simulink subsystem "pitchYawInnerLoop"  (R2026a)
settings: Solver=VariableStepAuto
values from neighbouring files (symbols this model uses):
  innerLoopParams = 180.0    [controllerParams.sldd]
libraries: slctrl_autotuning x1
settings Model: DataDictionary=controllerParams.sldd  EnableAccessToBaseWorkspace=off  Creator=maxhu  LastModifiedBy=maxhu

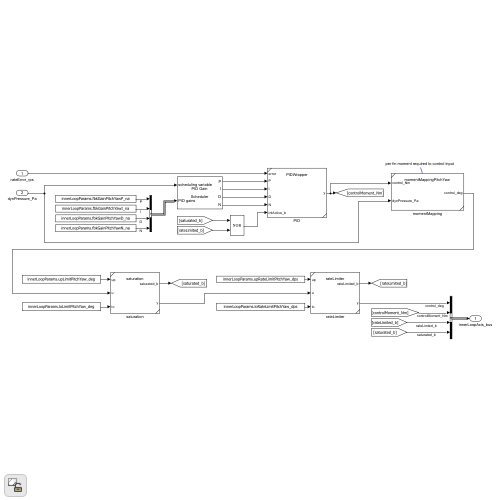
[thumbnail: Simulink's stored preview of the top-level diagram]
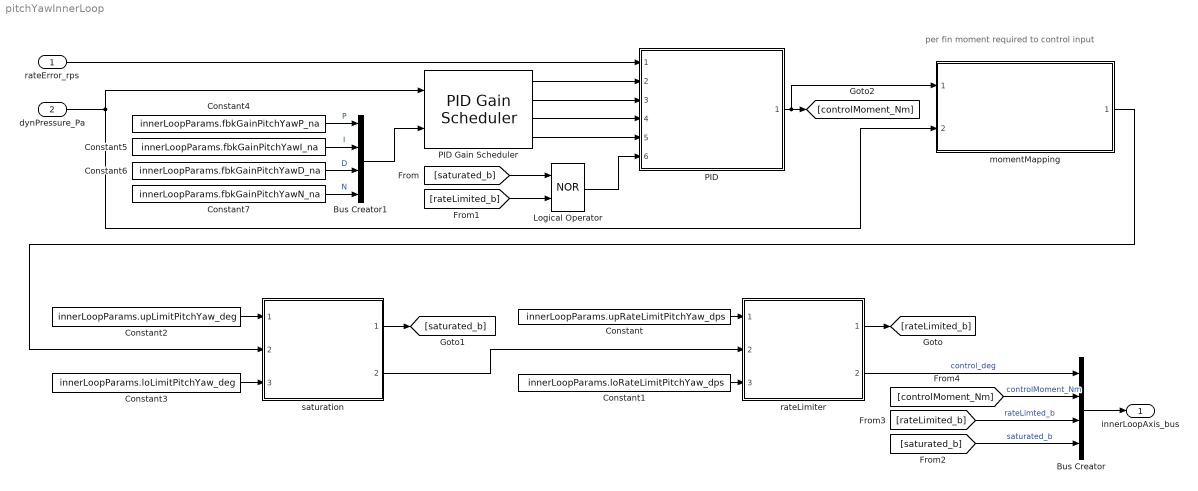
== system pitchYawInnerLoop ==
  note: per fin moment required to control input
  rateError_rps : Inport
  dynPressure_Pa : Inport  Port=2
  Bus Creator : BusCreator  Inputs=4
  Bus Creator1 : BusCreator  Inputs=4
  Constant : Constant  Value=innerLoopParams.upRateLimitPitchYaw_dps
  Constant1 : Constant  Value=innerLoopParams.loRateLimitPitchYaw_dps
  Constant2 : Constant  Value=innerLoopParams.upLimitPitchYaw_deg
  Constant3 : Constant  Value=innerLoopParams.loLimitPitchYaw_deg
  Constant4 : Constant  Value=innerLoopParams.fbkGainPitchYawP_na
  Constant5 : Constant  Value=innerLoopParams.fbkGainPitchYawI_na
  Constant6 : Constant  Value=innerLoopParams.fbkGainPitchYawD_na
  Constant7 : Constant  Value=innerLoopParams.fbkGainPitchYawN_na
  Logical Operator : Logic  Operator=NOR  AllPortsSameDT=off  OutDataTypeStr=boolean
  PID : Subsystem  ReferencedSubsystem=PIDWrapper
  PID Gain Scheduler : slctrl_autotuning/PID Gain Scheduler  InstantiateOnLoad=on  ControllerType=PIDN  BPsInGainArray=off  UseTwoSchedulingVariables=off  GainArrayBreakpoints=innerLoopParams.fbkGainBreakpoints_Pa  GainArrayBreakpoints2=[1 2 3 4]  NumBreakpoints=3  NumBreakpoints2=4  UseExternalBreakpoints=off  GainSourceMethod=Input to block  StoreGainsPParamName=PGain  StoreGainsIParamName=IGain  StoreGainsDParamName=DGain  StoreGainsNParamName=NGain  BlockDataType=Double  PGainLookUpMeth=Interpolation-Use End Values  IGainLookUpMeth=Interpolation-Use End Values  DGainLookUpMeth=Interpolation-Use End Values  NGainLookUpMeth=Interpolation-Use End Values  DoSatur=off  BreakpointSourceLookupVariant=InternalBPs  GainSourceVariant=DataStoreMemory  BreakpointSourceVariant=InternalBPs  PGainVariant=Enabled  IGainVariant=Enabled  DGainVariant=Enabled  NGainVariant=Enabled
      settings: LibrarySourceBlock=slctrlblks/Autotuning/PID Gain Scheduler
  momentMapping : Subsystem  ReferencedSubsystem=momentMappingPitchYaw
  rateLimiter : Subsystem  ReferencedSubsystem=rateLimiter
  saturation : Subsystem  ReferencedSubsystem=saturation
  innerLoopAxis_bus : Outport
  wires:
  PID Gain Scheduler/1 -> PID/2
  Logical Operator/1 -> PID/6
  PID Gain Scheduler/2 -> PID/3
  PID Gain Scheduler/3 -> PID/4
  rateError_rps/1 -> PID/1
  PID Gain Scheduler/4 -> PID/5
  [saturated_b] -> Logical Operator/1
  dynPressure_Pa/1 -> momentMapping/2, PID Gain Scheduler/1
  PID/1 -> [controlMoment_Nm], momentMapping/1
  Bus Creator1/1 -> PID Gain Scheduler/2
  rateLimiter/1 -> [rateLimited_b]
  Constant/1 -> rateLimiter/1
  saturation/2 -> rateLimiter/2
  Constant3/1 -> saturation/3
  saturation/1 -> [saturated_b]
  Bus Creator/1 -> innerLoopAxis_bus/1
  Constant1/1 -> rateLimiter/3
  [saturated_b] -> Bus Creator/4  "saturated_b"
  [rateLimited_b] -> Bus Creator/3  "rateLimted_b"
  rateLimiter/2 -> Bus Creator/1  "control_deg"
  Constant2/1 -> saturation/1
  momentMapping/1 -> saturation/2
  [controlMoment_Nm] -> Bus Creator/2  "controlMoment_Nm"
  [rateLimited_b] -> Logical Operator/2
  Constant4/1 -> Bus Creator1/1  "P"
  Constant5/1 -> Bus Creator1/2  "I"
  Constant6/1 -> Bus Creator1/3  "D"
  Constant7/1 -> Bus Creator1/4  "N"
